simulink model "kalmanbucy"  (Simulink 6.1)
settings: Solver=ode45  StartTime=0.0  StopTime=10.0  RelTol=1e-3
values from neighbouring files (symbols this model uses):
  A = [-1.4576   -0.3369    1.0503    3.7815 ... (first row only)    [runkalmanbucy.m]
  A1 = A    [runkalmanbucy.m]
  B = [-0.1072         0 ... (first row only)    [runkalmanbucy.m]
  B1 = B    [runkalmanbucy.m]
  C = [0.1685   -0.9595   -0.0755   -0.3771]    [runkalmanbucy.m]
  C1 = C    [runkalmanbucy.m]
  D = [0 0]    [runkalmanbucy.m]
  D1 = D    (= 0)    [runkalmanbucy.m]
  P1 = 10*eye(4)    [runkalmanbucy.m]
  Q = diag([0.5^2 0.2^2 0.3^2 0.5^2])    [runkalmanbucy.m]
  Q1 = Q    [runkalmanbucy.m]
  R = 1    [runkalmanbucy.m]
  R1 = R    (= 1)    [runkalmanbucy.m]
  x0 = [-1.7073 ... (first row only)    [runkalmanbucy.m]
  x1 = zeros(4,1)    [runkalmanbucy.m]
settings Model: Creator=fo1521  LastModifiedBy=fo1521
settings OptimizationCC: InlineInvariantSignals=off
settings DebuggingCC: SignalResolutionControl=UseLocalSettings  MultiTaskDSMMsg=error
settings GRTTargetCC: TargetFcnLib=ansi_tfl_table_tmw.mat

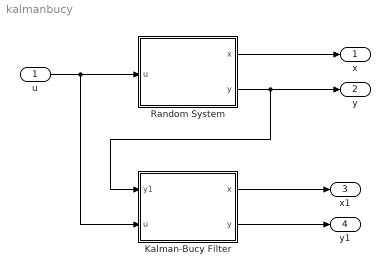
== system kalmanbucy ==
  u : Inport  Port=1  LatchInput=off
  Kalman-Bucy Filter : Subsystem  mask{x0=x1, P0=P1, A=A1, B=B1, C=C1, D=D1, Q=Q1, R=R1}
      mask Display:
      | port_label('input',1,'y')
      | port_label('input',2,'u')
      | port_label('output',1,'x')
      | port_label('output',2,'y')
      | disp(sprintf('Kalman-Bucy\n Filter'))
  Random System : Subsystem  mask{x0=x0, A=A, B=B, C=C, D=D, Q=sqrtm(Q), R=sqrtm(R)}
      mask Display:
      | port_label('input',1,'u')
      | port_label('output',1,'x')
      | port_label('output',2,'y')
      | disp(sprintf('Gassian\n Process'))
  x : Outport
  y : Outport  Port=2
  x1 : Outport  Port=3
  y1 : Outport  Port=4
  wires:
  Random System/1(x) -> x/1
  Random System/2(y) -> Kalman-Bucy Filter/1(y1), y/1
  Kalman-Bucy Filter/1(x) -> x1/1
  Kalman-Bucy Filter/2(y) -> y1/1
  u/1 -> Random System/1(u), Kalman-Bucy Filter/2(u)

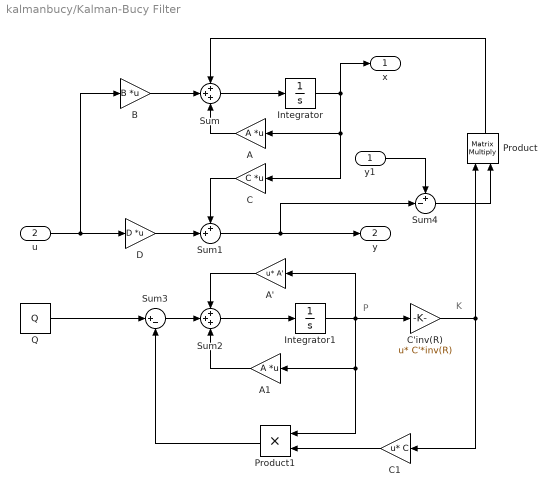
== system kalmanbucy/Kalman-Bucy Filter ==
  note: K
  note: P
  y1 : Inport  Port=1  LatchInput=off
  u : Inport  Port=2  PortDimensions=size(B,2)  LatchInput=off
  A : Gain  Orientation=left  Gain=A  Multiplication=Matrix(K*u)
  A' : Gain  Orientation=left  Gain=A'  Multiplication=Matrix(u*K)
  A1 : Gain  Orientation=left  Gain=A  Multiplication=Matrix(K*u)
  B : Gain  Gain=B  Multiplication=Matrix(K*u)
  C : Gain  Orientation=left  Gain=C  Multiplication=Matrix(K*u)
  C'inv(R) : Gain  Gain=C'*inv(R)  Multiplication=Matrix(u*K)
  C1 : Gain  Orientation=left  Gain=C  Multiplication=Matrix(u*K)
  D : Gain  Gain=D  Multiplication=Matrix(K*u)
  Integrator : Integrator  InitialCondition=x0
  Integrator1 : Integrator  InitialCondition=P0
  Product : Product  Orientation=up  Multiplication=Matrix(*)  RndMeth=Zero
  Product1 : Product  Orientation=left  RndMeth=Zero
  Q : Constant  Value=Q
  Sum : Sum  Inputs=+++
  Sum1 : Sum  Inputs=++|
  Sum2 : Sum  Inputs=+++
  Sum3 : Sum  Inputs=|+-
  Sum4 : Sum  Inputs=+-|
  x : Outport
  y : Outport  Port=2
  wires:
  Sum1/1 -> y/1, Sum4/2
  D/1 -> Sum1/2
  C/1 -> Sum1/1
  B/1 -> Sum/2
  A/1 -> Sum/3
  Integrator/1 -> x/1, C/1, A/1
  Sum/1 -> Integrator/1
  u/1 -> D/1, B/1
  Sum2/1 -> Integrator1/1
  Integrator1/1 -> A'/1, C'inv(R)/1, A1/1, Product1/1
  A1/1 -> Sum2/3
  A'/1 -> Sum2/1
  Q/1 -> Sum3/1
  Sum3/1 -> Sum2/2
  y1/1 -> Sum4/1
  Product/1 -> Sum/1
  C'inv(R)/1 -> C1/1, Product/1
  Product1/1 -> Sum3/2
  C1/1 -> Product1/2
  Sum4/1 -> Product/2

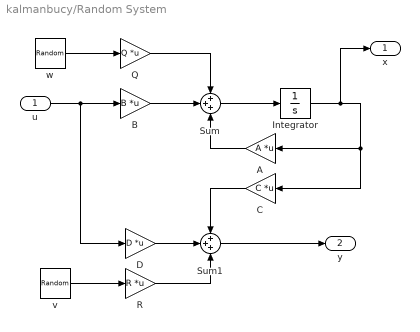
== system kalmanbucy/Random System ==
  u : Inport  Port=1  PortDimensions=size(B,2)  LatchInput=off
  A : Gain  Orientation=left  Gain=A  Multiplication=Matrix(K*u)
  B : Gain  Gain=B  Multiplication=Matrix(K*u)
  C : Gain  Orientation=left  Gain=C  Multiplication=Matrix(K*u)
  D : Gain  Gain=D  Multiplication=Matrix(K*u)
  Integrator : Integrator  InitialCondition=x0
  Q : Gain  Gain=Q  Multiplication=Matrix(K*u)
  R : Gain  Gain=R  Multiplication=Matrix(K*u)
  Sum : Sum  Inputs=+++
  Sum1 : Sum  Inputs=+++
  v : RandomNumber  Mean=zeros(size(R,1),1)  Variance=ones(size(R,1),1)  SampleTime=0
  w : RandomNumber  Mean=zeros(numel(x0),1)  Variance=ones(numel(x0),1)  SampleTime=0
  x : Outport
  y : Outport  Port=2
  wires:
  Sum/1 -> Integrator/1
  Integrator/1 -> A/1, C/1, x/1
  A/1 -> Sum/3
  B/1 -> Sum/2
  u/1 -> B/1, D/1
  w/1 -> Q/1
  Q/1 -> Sum/1
  C/1 -> Sum1/1
  D/1 -> Sum1/2
  v/1 -> R/1
  R/1 -> Sum1/3
  Sum1/1 -> y/1
